simulink model "IPCBlockTetheredExampleTest"  (R2019a)
settings: Solver=VariableStepAuto  StartTime=0.0  StopTime=inf  RelTol=1e-3
settings Model: EnablePacing=on  Creator=wuyuanyi  LastModifiedBy=wuyuanyi

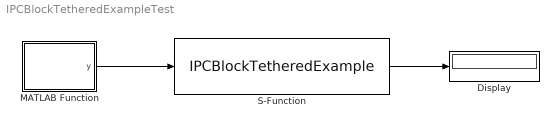
== system IPCBlockTetheredExampleTest ==
  Display : Display
  MATLAB Function : MATLAB Function  TreatAsAtomicUnit=on
  S-Function : S-Function  FunctionName=IPCBlockTetheredExample  SFunctionDeploymentMode=off  EnableBusSupport=off
  wires:
  MATLAB Function/1(y) -> S-Function/1
  S-Function/1 -> Display/1

== matlab function IPCBlockTetheredExampleTest/MATLAB Function ==
  data: y output
function y = fcn()

y = rand(1,1);
